simulink model "bird"  (R2022a)
settings: Solver=VariableStepAuto  StartTime=0.0  StopTime=250.0  RelTol=1e-3
settings Model: PacingRate=1000  Creator=violet_in_summer  LastModifiedBy=violet_in_summer

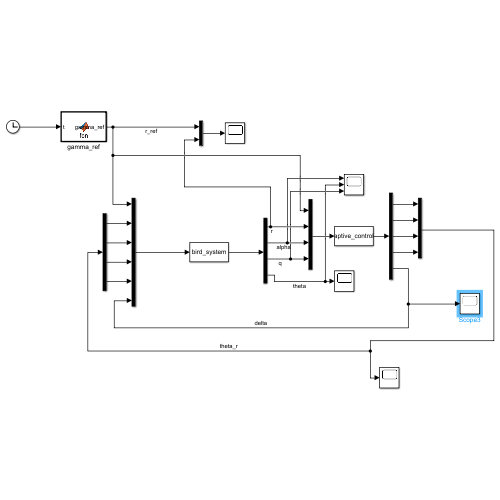
[thumbnail: Simulink's stored preview of the top-level diagram]
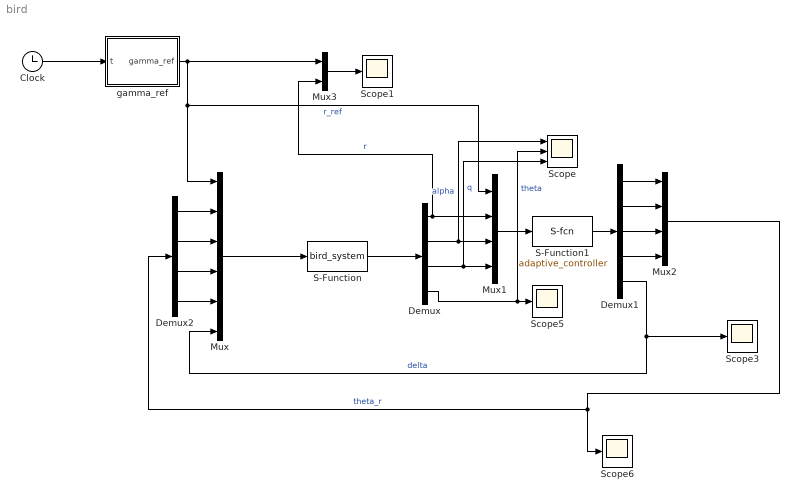
== system bird ==
  Clock : Clock
  Demux : Demux
  Demux1 : Demux  Outputs=5
  Demux2 : Demux
  Mux : Mux  Inputs=6
  Mux1 : Mux
  Mux2 : Mux
  Mux3 : Mux  Inputs=2
  S-Function : S-Function  FunctionName=bird_system  Parameters=para  SFunctionDeploymentMode=off  EnableBusSupport=off
  S-Function1 : S-Function  FunctionName=adaptive_controller  Parameters=para  SFunctionDeploymentMode=off  EnableBusSupport=off
  Scope : Scope  NumInputPorts=3
  Scope{1,3,5..6} (4 alike) : Scope
  gamma_ref : MATLAB Function  TreatAsAtomicUnit=on
  wires:
  Mux/1 -> S-Function/1
  S-Function/1 -> Demux/1
  Mux1/1 -> S-Function1/1
  S-Function1/1 -> Demux1/1
  Clock/1 -> gamma_ref/1(t)
  gamma_ref/1(gamma_ref) -> Mux3/1, Mux1/1, Mux/1  "r_ref"
  Demux1/1 -> Mux2/1
  Demux1/2 -> Mux2/2
  Demux1/3 -> Mux2/3
  Demux1/4 -> Mux2/4
  Demux1/5 -> Scope3/1, Mux/6  "delta"
  Demux/1 -> Mux3/2, Mux1/2  "r"
  Demux/2 -> Mux1/3, Scope/1  "alpha"
  Demux/3 -> Mux1/4, Scope/3  "q"
  Mux2/1 -> Scope6/1, Demux2/1  "theta_r"
  Demux2/1 -> Mux/2
  Demux2/2 -> Mux/3
  Demux2/3 -> Mux/4
  Demux2/4 -> Mux/5
  Demux/4 -> Scope/2, Scope5/1  "theta"
  Mux3/1 -> Scope1/1

== matlab function bird/gamma_ref ==
  data: t input; gamma_ref output
function gamma_ref = fcn(t)
if (t>=0) && (t<20)
    gamma_ref = 0;
elseif (t>=20) && (t<50)
    gamma_ref = 10;
elseif (t>=50) && (t<80)
    gamma_ref = 5;
elseif (t>=80) && (t<120)
    gamma_ref = -3;
elseif (t>=120) && (t<160)
    gamma_ref = 4;
else
    gamma_ref = 0;
end
